simulink model "Controller1"  (R2022b)
settings: Solver=ode4  StartTime=0.0  StopTime=40  FixedStep=0.00001  RelTol=1e-3
settings Model: Creator=Sahil Gaurkar  LastModifiedBy=Sahil Gaurkar

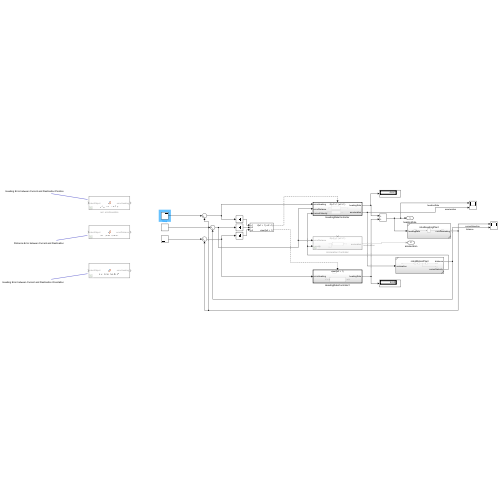
[thumbnail: Simulink's stored preview of the top-level diagram]
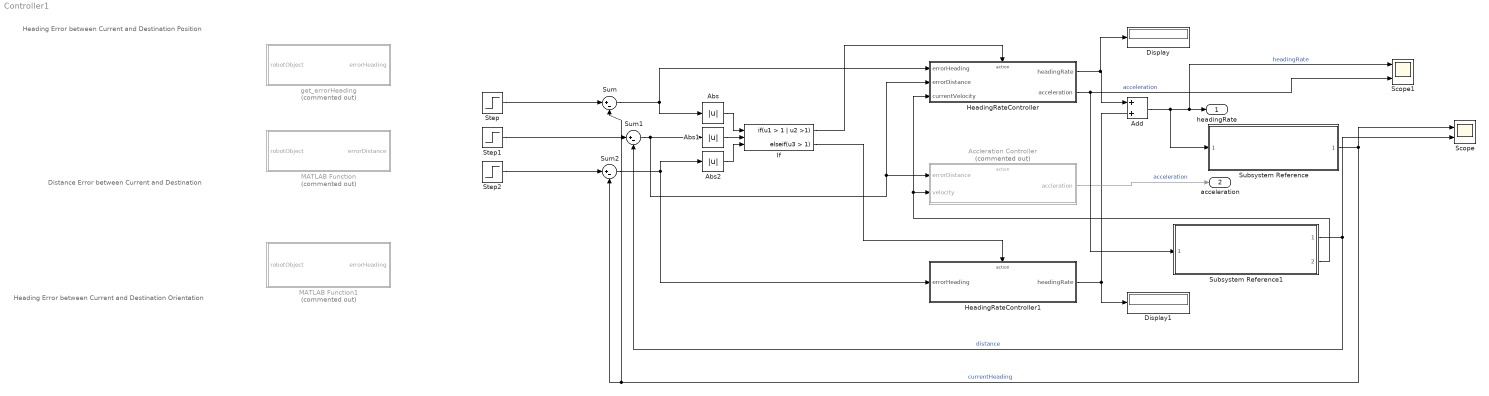
== system Controller1 ==
  note: Heading Error between Current and Destination Orientation
  note: Heading Error between Current and Destination Position
  note: Distance Error between Current and Destination
  Abs : Abs  SaturateOnIntegerOverflow=off
  Abs1 : Abs  SaturateOnIntegerOverflow=off
  Abs2 : Abs  SaturateOnIntegerOverflow=off
  Accleration Controller : Subsystem  Commented=on  TreatAsAtomicUnit=on
  Add : Sum
  Display : Display
  Display1 : Display
  HeadingRateController : Subsystem  TreatAsAtomicUnit=on
  HeadingRateController1 : Subsystem  TreatAsAtomicUnit=on
  If : If  NumInputs=3  IfExpression=u1 > 1 | u2 >1  ElseIfExpressions=u3 > 1  ShowElse=off
  MATLAB Function : MATLAB Function  Commented=on  TreatAsAtomicUnit=on
  MATLAB Function1 : MATLAB Function  Commented=on  TreatAsAtomicUnit=on
  Scope : Scope  NumInputPorts=2
  Scope1 : Scope  NumInputPorts=2
  Step : Step  After=90  SampleTime=0
  Step1 : Step  After=1000  SampleTime=0
  Step2 : Step  After=180  SampleTime=0
  Subsystem Reference : Subsystem  ReferencedSubsystem=robotHeadingPlant
  Subsystem Reference1 : Subsystem  ReferencedSubsystem=robotMotionPlant
  Sum : Sum  Inputs=|+-
  Sum1 : Sum  Inputs=|+-
  Sum2 : Sum  Inputs=|+-
  get_errorHeading : MATLAB Function  Commented=on  TreatAsAtomicUnit=on
  headingRate : Outport
  acceleration : Outport  Port=2
  wires:
  HeadingRateController/1(headingRate) -> Display/1, Add/1
  Add/1 -> Subsystem Reference/1, Scope1/1, headingRate/1  "headingRate"
  If/1 -> HeadingRateController/Action
  HeadingRateController1/1(headingRate) -> Display1/1, Add/2
  Accleration Controller/1(accleration) -> acceleration/1  "acceleration"
  Step/1 -> Sum/1
  Sum/1 -> HeadingRateController/1(errorHeading), Abs/1
  Step2/1 -> Sum2/1
  Step1/1 -> Sum1/1
  Sum1/1 -> HeadingRateController/2(errorDistance), Accleration Controller/1(errorDistance), Abs1/1
  Sum2/1 -> HeadingRateController1/1(errorHeading), Abs2/1
  Subsystem Reference/1 -> Sum2/2, Sum/2, Scope/1  "currentHeading"
  Subsystem Reference1/1 -> Scope/2, Sum1/2  "distance"
  Subsystem Reference1/2 -> HeadingRateController/3(currentVelocity), Accleration Controller/2(velocity)
  Abs/1 -> If/1
  Abs1/1 -> If/2
  Abs2/1 -> If/3
  If/2 -> HeadingRateController1/Action
  HeadingRateController/2(acceleration) -> Subsystem Reference1/1, Scope1/2  "acceleration"

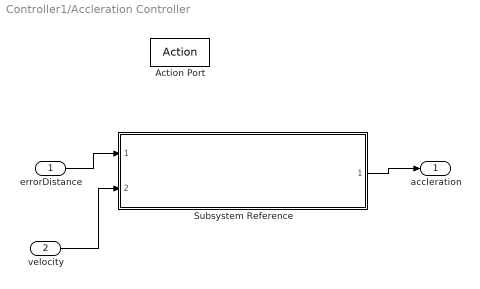
== system Controller1/Accleration Controller ==
  errorDistance : Inport
  velocity : Inport  Port=2
  Action Port : ActionPort  ActionPortLabel=if(u1 > 1 | u2 >1)
  Subsystem Reference : Subsystem  ReferencedSubsystem=AcclerationController
  accleration : Outport
  wires:
  errorDistance/1 -> Subsystem Reference/1
  Subsystem Reference/1 -> accleration/1
  velocity/1 -> Subsystem Reference/2

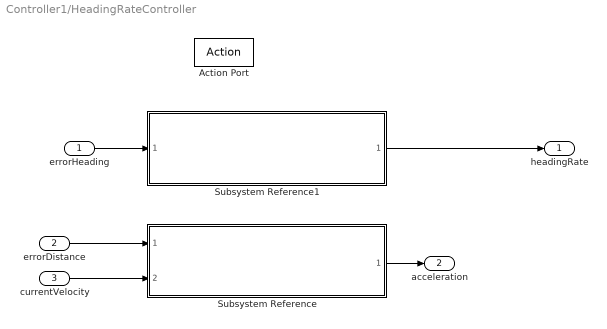
== system Controller1/HeadingRateController ==
  errorHeading : Inport
  errorDistance : Inport  Port=2
  currentVelocity : Inport  Port=3
  Action Port : ActionPort  ActionPortLabel=if(u1 > 1 | u2 >1)
  Subsystem Reference : Subsystem  ReferencedSubsystem=AcclerationController
  Subsystem Reference1 : Subsystem  ReferencedSubsystem=HeadingRateController
  headingRate : Outport
  acceleration : Outport  Port=2
  wires:
  errorHeading/1 -> Subsystem Reference1/1
  currentVelocity/1 -> Subsystem Reference/2
  errorDistance/1 -> Subsystem Reference/1
  Subsystem Reference/1 -> acceleration/1
  Subsystem Reference1/1 -> headingRate/1

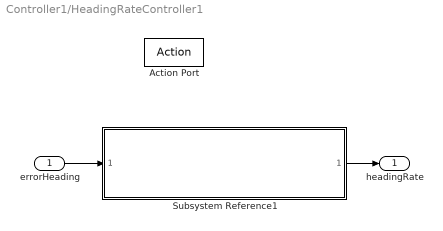
== system Controller1/HeadingRateController1 ==
  errorHeading : Inport
  Action Port : ActionPort  ActionPortLabel=elseif(u3 > 1)
  Subsystem Reference1 : Subsystem  ReferencedSubsystem=HeadingRateController
  headingRate : Outport
  wires:
  errorHeading/1 -> Subsystem Reference1/1
  Subsystem Reference1/1 -> headingRate/1

== matlab function Controller1/MATLAB Function ==
  data: robotObject input; errorDistance output
function errorDistance = get_errorDistance(robotObject)

errorDistance = pdist2(robotObject.destinationPose(1:2), robotObject.currentPose(1:2), 'euclidean');

end

== matlab function Controller1/MATLAB Function1 ==
  data: robotObject input; errorHeading output
function errorHeading = get_errorHeading1(robotObject)

errorHeading = robotObject.destinationPose(3) - robotObject.currentPose(3);

end

== matlab function Controller1/get_errorHeading ==
  data: robotObject input; errorHeading output
function errorHeading = get_errorHeading(robotObject)
errorHeading = atan2d(robotObject.destinationPose(2) - robotObject.currentPose(2), robotObject.destinationPose(1) - robotObject.currentPose(1)) - robotObject.currentPose(3);
end
